simulink model "DenemeDcMotorwithFeedback"  (R2016a)
settings: Solver=VariableStepAuto  StartTime=0.0  StopTime=2  RelTol=1e-3
libraries: powerlib x12, simulink x2, electricdrivelib x1
settings Model: Creator=M.Cihan  LastModifiedBy=M.Cihan

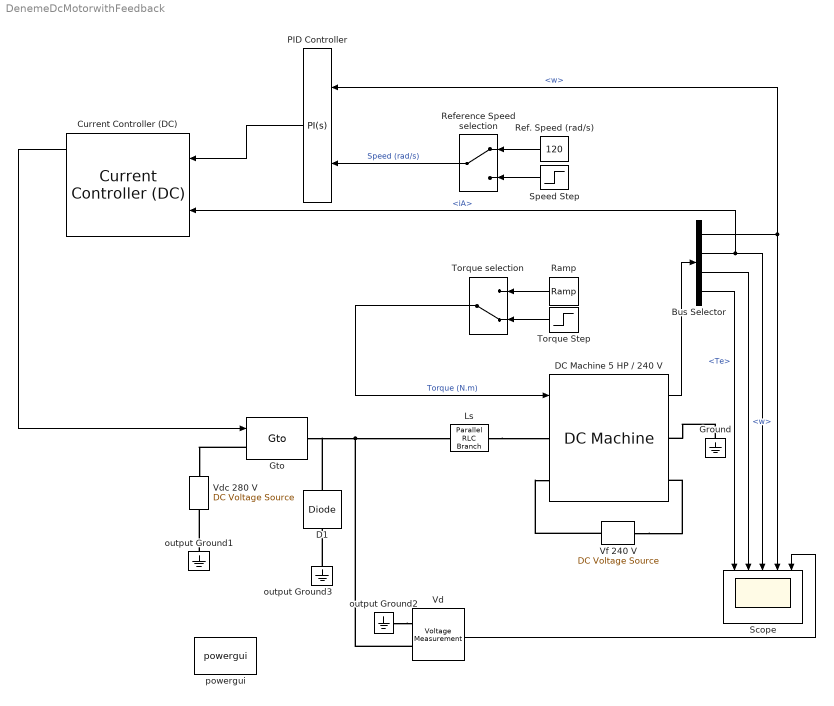
== system DenemeDcMotorwithFeedback ==
  Bus Selector : BusSelector  OutputSignals=w,iA,w,Te
  Current Controller (DC) : electricdrivelib/Fundamental Drive Blocks/Current Controller (DC)  OverrideUsingVariant=Chopper_detailed_1q  driveType=Chopper based  detailLevel=Detailed  numQuadChop=1  numQuadRect=2  Pb=5*746  Vb=280  Kp=1  Ki=1  fci=500  F=5e3  lim=[20, 160]  sampling=20e-6  Ts=1e-6
  D1 : powerlib/Power Electronics/Diode  Ron=0.05  Lon=0  Vf=0.7  IC=0  UseSnubber=off  Rs=Inf  Cs=0.1e-6  Measurements=off
  DC Machine 5 HP / 240 V : powerlib/Machines/DC Machine  PresetModel=No  MechanicalLoad=Torque TL  FieldType=Wound  ShowDetailedParameters=on  MeasurementBus=on  RLa="[ 0.5  0.01]"  RLf="[ 240  120]"  Laf=1.23  MachineConstant=Torque constant (N.m/A)  Ke=1.8  Kt=1.8  J=0.05  Bm=0.02  Tf=0  w0=0.1  Ifinit=0  TsPowergui=0  TsBlock=-1
  Ground : powerlib/Elements/Ground  LConnTagsString=a
  Gto : powerlib/Power Electronics/Gto  Ron=0.05  Lon=0  Vf=1  Tf=1e-6  Tt=1e-6  IC=0  Rs=1e4  Cs=inf  Measurements=off
      settings: AttributesFormatString=\n
  Ls : powerlib/Elements/Parallel RLC Branch  LConnTagsString=a  RConnTagsString=__new0  BranchType=L  Resistance=[]  Inductance=10e-03  SetiL0=off  InitialCurrent=0  Capacitance=[]  Setx0=off  InitialVoltage=0  Measurements=None
  PID Controller : simulink/Continuous/PID Controller  Controller=PI  TimeDomain=Continuous-time  SampleTime=-1  IntegratorMethod=Forward Euler  FilterMethod=Forward Euler  Form=Ideal  UseFilter=on  ControllerParametersSource=internal  P=1.6  I=16  D=0  N=100  InitialConditionSource=external  InitialConditionForIntegrator=0  InitialConditionForFilter=0  ExternalReset=none  LimitOutput=on  UpperSaturationLimit=30  LowerSaturationLimit=-30  LinearizeAsGain=on  AntiWindupMode=none  Kb=1  TrackingMode=off  Kt=1  PParamMin=[]  PParamMax=[]  IParamMin=[]  IParamMax=[]  DParamMin=[]  DParamMax=[]  NParamMin=[]  NParamMax=[]  KbParamMin=[]  KbParamMax=[]  KtParamMin=[]  KtParamMax=[]  POutMin=[]  POutMax=[]  IOutMin=[]  IOutMax=[]  DOutMin=[]  DOutMax=[]  NOutMin=[]  NOutMax=[]  KbOutMin=[]  KbOutMax=[]  KtOutMin=[]  KtOutMax=[]  IntegratorOutMin=[]  IntegratorOutMax=[]  FilterOutMin=[]  FilterOutMax=[]  SumOutMin=[]  SumOutMax=[]  SumI1OutMin=[]  SumI1OutMax=[]  SumI2OutMin=[]  SumI2OutMax=[]  SumI3OutMin=[]  SumI3OutMax=[]  SumDOutMin=[]  SumDOutMax=[]  SaturationOutMin=[]  SaturationOutMax=[]  IntegratorContinuousStateAttributes=''  IntegratorStateMustResolveToSignalObject=off  IntegratorRTWStateStorageClass=Auto  FilterContinuousStateAttributes=''  FilterStateMustResolveToSignalObject=off  FilterRTWStateStorageClass=Auto  DifferentiatorICPrevScaledInput=0  DifferentiatorOutMin=[]  DifferentiatorOutMax=[]
  Ramp : simulink/Sources/Ramp  slope=50  start=1  X0=10
  Ref. Speed (rad/s) : Constant  Value=120
  Reference Speed selection : ManualSwitch
  Scope : Scope  NumInputPorts=5
  Speed Step : Step  Time=0.4  Before=120  After=160  SampleTime=0
  Torque selection : ManualSwitch  CurrentSetting=0
  Torque Step : Step  Time=0.5  After=20  SampleTime=0
  Vd : powerlib/Measurements/Voltage Measurement  Tag=PoWeRsYsTeMmEaSuReMeNt  PhasorSimulation=off  OutputType=Magnitude  PSBequivalent=0
  "Vdc 280 V " : powerlib/Electrical Sources/DC Voltage Source  Description=source block  Amplitude=280  Measurements=Voltage
      settings: AttributesFormatString=\n
  Vf 240 V : powerlib/Electrical Sources/DC Voltage Source  Description=source block  Amplitude=240  Measurements=None
      settings: AttributesFormatString=\n
  output Ground1 : powerlib/Elements/Ground  LConnTagsString=a
  output Ground2 : powerlib/Elements/Ground  LConnTagsString=a
  output Ground3 : powerlib/Elements/Ground  LConnTagsString=a
  powergui : powerlib/powergui  Priority=1  SimulationMode=Continuous  SolverType=Tustin/Backward Euler (TBE)  SampleTime=50e-6  frequency=60  SPID=on  DisableSnubberDevices=on  DisableRonSwitches=off  DisableVfSwitches=off  SwTol=0  DisplayEquations=off  Interpol=off  ExternalGateDelay=off  methode=off  Ts=10  FunctionMessages=off  echomessages=off  HookPort=off  EnableUseOfTLC=off  x0status=blocks  frequencyindice=0  Pbase=100e6  ErrMax=1e-4  Iterations=50  UnitsV=kV  UnitsW=MW  buscounter=0  RestoreLinks=warning  ResistiveCurrentMeasurement=off  Frange=[0:2:500]  Ylog=off  Xlog=on  ShowGrid=off  save=off  variable=ZData  structure=0  ZoomFFT=off  StartTime=0.0  cycles=1  DisplayStyle=1  fundamental=60  FreqAxis=off  MaxFrequency=1000  frequencyindicesteady=1  RmsSteady=1  display=off
  wires:
  DC Machine 5 HP / 240 V/1 -> Bus Selector/1
  Ramp/1 -> Torque selection/1
  Torque Step/1 -> Torque selection/2
  Torque selection/1 -> DC Machine 5 HP / 240 V/1  "Torque (N.m)"
  Bus Selector/4 -> Scope/1  "<Te>"
  Bus Selector/3 -> Scope/2  "<w>"
  Bus Selector/2 -> Current Controller (DC)/1, Scope/3  "<iA>"
  Bus Selector/1 -> PID Controller/1, Scope/4  "<w>"
  Vd/1 -> Scope/5
  Ref. Speed (rad/s)/1 -> Reference Speed selection/1
  Speed Step/1 -> Reference Speed selection/2
  Reference Speed selection/1 -> PID Controller/2  "Speed (rad/s)"
  PID Controller/1 -> Current Controller (DC)/2
  Current Controller (DC)/4 -> Gto/1
  connections:
  Vf 240 V/RConn1 -- DC Machine 5 HP / 240 V/LConn2
  Vf 240 V/LConn1 -- DC Machine 5 HP / 240 V/RConn2
  Ls/RConn1 -- DC Machine 5 HP / 240 V/LConn1
  Ground/LConn1 -- DC Machine 5 HP / 240 V/RConn1
  output Ground1/LConn1 -- "Vdc 280 V "/LConn1
  Vd/LConn1 -- D1/RConn1 -- Gto/RConn1 -- Ls/LConn1
  output Ground2/LConn1 -- Vd/LConn2
  Gto/LConn1 -- "Vdc 280 V "/RConn1
  output Ground3/LConn1 -- D1/LConn1
